simulink model "QAMGainControlV1"  (R2023a)
settings: Solver=FixedStepAuto  StartTime=0.0  StopTime=tStop  FixedStep=tStepSize  MaxStep=tStepSize  RelTol=1e-3
settings Model: Creator=athmajanvivekananthan  LastModifiedBy=athmajanvivekananthan
settings DataIOCC: ReturnWorkspaceOutputs=off

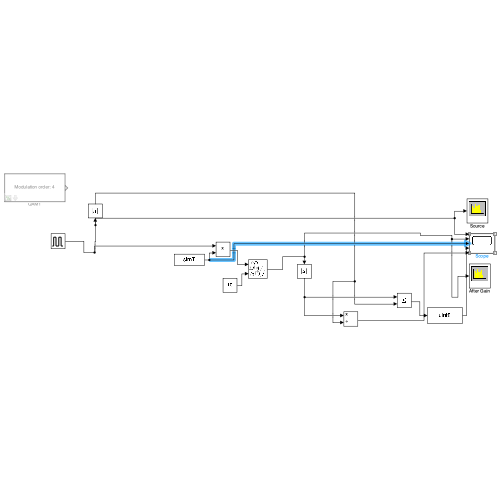
[thumbnail: Simulink's stored preview of the top-level diagram]
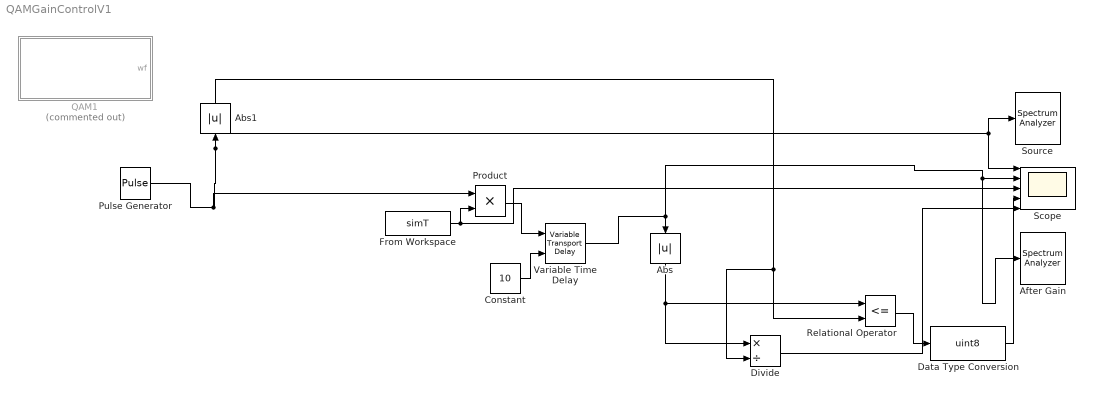
== system QAMGainControlV1 ==
  Abs : Abs  SaturateOnIntegerOverflow=off
  Abs1 : Abs  SaturateOnIntegerOverflow=off
  After Gain : SpectrumAnalyzer  WindowPosition=[35.000000,138.000000,800.000000,500.000000,]  Visible=on  ScopeFrameLocation=window  Span=1000  StartFrequency=-500  StopFrequency=500  YLimits=[-79.19848851,29.96144614]  ColorLimits=[-80 20]
  Constant : Constant  Value=10
  Data Type Conversion : DataTypeConversion  OutDataTypeStr=uint8  SaturateOnIntegerOverflow=off  RndMeth=Floor
  Divide : Product  Inputs=*/
  From Workspace : FromWorkspace  VariableName=simT  OutDataTypeStr=double
  Product : Product
  Pulse Generator : DiscretePulseGenerator  PulseType=Time based  Period=1  PulseWidth=50
  QAM1 : MATLAB Function  Tag=BlockGeneratedWWGApp  Commented=on  TreatAsAtomicUnit=on  SystemSampleTime=0.0010000000000000000208  mask(QAM Waveform Generator){nsamps=1, OutputAfterFinalValue=Cyclic repetition}
      mask prompts: nsamps "Samples per frame:"; OutputAfterFinalValue "Form output after final data value by:"
      mask init:
      | %% Generating QAM waveform
      | % QAM configuration
      | M = 4; 	 % Modulation order
      | % input bit source:
      | in = randi([0, 1], 60000, 1);
      | 
      | % Generation
      | waveform = qammod(in, M, 'gray', 'InputType', 'bit', 'UnitAveragePower', true);
      | 
      | Fs = 1000; 								 % Specify the sample rate of the waveform in Hz
      | 
      | %% Configuring block: update parameters and UserData
      | % Get current block
      | thisBlock = gcb;
      | 
      | % Set info parameters
      | maskHandle = Simulink.Mask.get(thisBlock);
      | textFsDialog = maskHandle.getDialogControl('textFs');
      | textFsDialog.Prompt = ['Waveform sample rate (Fs): ' num2str(Fs*1e-6,'%.9g') ' MHz'];
      | textWfLengthDialog = maskHandle.getDialogControl('textWFLength');
      | textWfLengthDialog.Prompt = ['Waveform length: ' num2str(length(waveform)) ' samples'];
      | 
      | % Set sample time of the block
      | set_param(thisBlock, 'SystemSampleTime', num2str(nsamps/Fs,'%.20g'));
      | 
      | % Update UserData
      | cfg.M = M;
      | cfg.Input = in;
      | outVar.WaveformConfig = cfg;
      | outVar.WaveformLength = length(waveform);
      | outVar.Fs = Fs;
      | set_param(thisBlock, 'UserData', outVar);
  Relational Operator : RelationalOperator  Operator=<=  OutDataTypeStr=boolean  RndMeth=Simplest  InputSameDT=off
  Scope : Scope  NumInputPorts=5
  Source : SpectrumAnalyzer  WindowPosition=[89.000000,144.000000,800.000000,500.000000,]  Visible=on  ScopeFrameLocation=window  Span=1000  StartFrequency=-500  StopFrequency=500  YLimits=[-72.40259764,34.45743035]  ColorLimits=[-80 20]
  Variable Time Delay : VariableTransportDelay  MaximumDelay=10
  wires:
  From Workspace/1 -> Scope/3, Product/2
  Product/1 -> Variable Time Delay/1
  Abs1/1 -> Divide/2, Relational Operator/2
  Variable Time Delay/1 -> After Gain/1, Scope/2, Abs/1
  Abs/1 -> Divide/1, Relational Operator/1
  Pulse Generator/1 -> Product/1, Abs1/1, Scope/1, Source/1
  Constant/1 -> Variable Time Delay/2
  Relational Operator/1 -> Data Type Conversion/1
  Data Type Conversion/1 -> Scope/4
  Divide/1 -> Scope/5

== matlab function QAMGainControlV1/QAM1 ==
  data: wf output; waveform parameter; nsamps parameter; OutputAfterFinalValue parameter
function wf = wfGenerator(waveform, nsamps, OutputAfterFinalValue)

% Create persistent variable
persistent src;

% Preallocate output
wf = complex(zeros(nsamps,size(waveform,2)));

if isempty(src)
    % Get action when signal ends
    if OutputAfterFinalValue == 1
        signalEndAction = 'Cyclic repetition';
    else
        signalEndAction = 'Set to zero';
    end
    
    % Initialize persistent dsp.SignalSource to get current frame
    src = dsp.SignalSource(waveform,nsamps,'SignalEndAction',signalEndAction);
end

% Extract current frame
wf(:,:) = src();

end
